simulink model "Final_project"  (R2020a)
settings: Solver=ode15s  StartTime=0.0  StopTime=1.6*3600  RelTol=1e-9
values from neighbouring files (symbols this model uses):
  a = (rp + ra)/2    (= 6781)    [final_project_data.m]
  alfa_earth = alfa_earth/alfa_tot    (= 0.0757575757576)    [final_project_data.m]
  alfa_mag = alfa_mag/alfa_tot    (= 0.0151515151515)    [final_project_data.m]
  alfa_sun = alfa_sun/alfa_tot    (= 0.454545454545)    [final_project_data.m]
  e = (ra - rp)/(rp + ra)    (= 0.00147470874502)    [final_project_data.m]
  F_e = 1358    [final_project_data.m]
  G = 6.67408e-11    [final_project_data.m]
  GK = lqr(A,B,Q,R)    [final_project_data.m]
  i = 51.6    [final_project_data.m]
  I_x = I(1)    [final_project_data.m]
  I_y = I(2)    [final_project_data.m]
  I_z = I(3)    [final_project_data.m]
  m_earth = 5.972e+24    [final_project_data.m]
  mu_e = 398600    [final_project_data.m]
  n = sqrt(mu_e/a^3)    [final_project_data.m]
  omega = 0    [final_project_data.m]
  omega_e = 2*pi/T_earth    (= 7.29212351699e-05)    [final_project_data.m]
  R_e = 6371    [final_project_data.m]
  RAAN = 0    [final_project_data.m]
undefined symbols (not defined in the file or in its folder): gm, gn, gvali, hm, hn, hvali
libraries: vrlib x4, simulink_extras x3
(part 1 of 2)
settings Model: SimulationMode=accelerator  Creator=dvdia  LastModifiedBy=dvdia
settings SolverCC: ZeroCrossAlgorithm=Adaptive
settings DebuggingCC: ReadBeforeWriteMsg=DisableAll  WriteAfterWriteMsg=DisableAll  WriteAfterReadMsg=DisableAll  IgnoredZcDiagnostic=none  MultiTaskDSMMsg=none
settings ModelReferenceCC: UpdateModelReferenceTargets=IfOutOfDate
settings SFSimCC: SFSimEcho=off  CustomCodeUndefinedFunction=UseInterfaceOnly

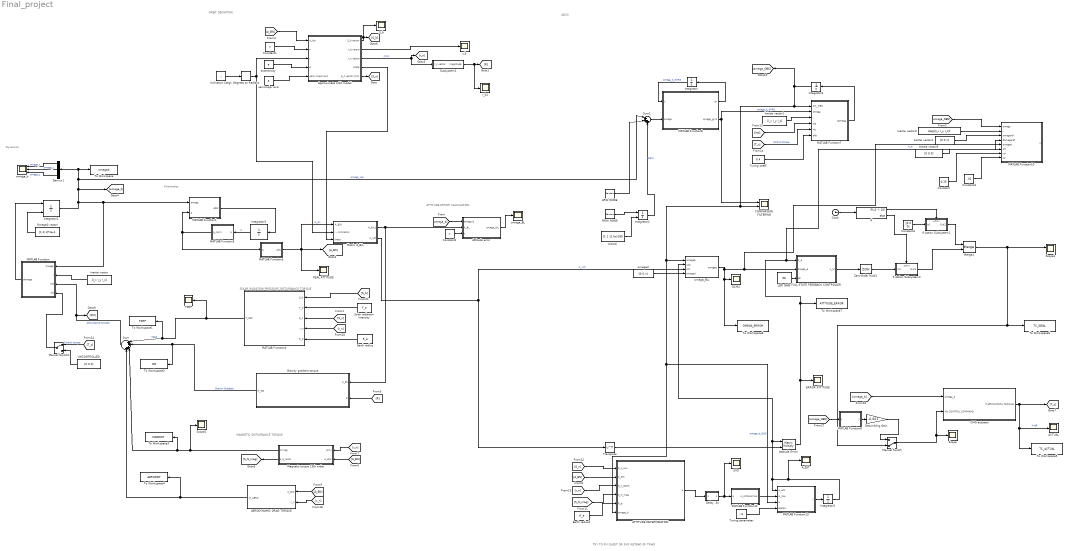
== system Final_project ==
  note: TRY TO FIX QUEST OR SVD INSTEAD OF TRIAD
  note: ADCS
  note: MAGNETIC DISTURBANCE TORQUE
  note: SOLAR RADIATION PRESSURE DISTURBANCE TORQUE
  note: ORBIT DEFINITION
  note: ATTITUDE ERROR CALCULATION
  note: Kinematics
  note: Dynamics
  ACTUAL : Scope
  AERODYNAMIC DRAG TORQUE : Subsystem
  ARW NOISE : RandomNumber  Variance=(0.0025*pi/180).^2.*[1 1 1]  SampleTime=1/10
  ATTITUDE DETERMINATION : Subsystem
  A_EST : Scope
  Approximate orbit model : Subsystem
  Attitude Errror : Product  Multiplication=Matrix(*)
  Attitude error : Subsystem
  CMG actuator : Subsystem
  COMPARISON FILTERING : Scope  NumInputPorts=2
  Clock : Clock
  Constant : Constant  Value=0.25
  Constant1 : Constant  Value=n
  Constant2 : Constant  Value=n
  Constant3 : Constant  Value=.01
  Constant4 : Constant  Value=[0 0 0]
  DCM2 : Scope
  Degrees to Radians : simulink_extras/Transformations/Degrees to Radians
  Delay .5s : Subsystem
  Demux1 : Demux  Outputs=3
  Detumbling Gain : Gain  Gain=-0.001
  ERROR ATTITUDE : Scope
  Earth radius : Constant  Value=R_e
  Earth radius1 : Constant  Value=R_e
  FULL STATE FEEDBACK CONTROLLER : MATLAB Function  TreatAsAtomicUnit=on
  Gravity gradient torque : Subsystem
  If : If  IfExpression=u1 < 10
  If Action Subsystem1 : Subsystem  TreatAsAtomicUnit=on
  If Action Subsystem2 : Subsystem  TreatAsAtomicUnit=on
  Inertia vector : Constant  Description=Inertia vector containing the inertias of the spacecraft in a PRINCIPAL AXIS REFERENCE SYSTEM  Value=[I_x I_y I_z]
  Inertia vector1 : Constant  Description=Inertia vector containing the inertias of the spacecraft in a PRINCIPAL AXIS REFERENCE SYSTEM  Value=[I_x I_y I_z]
  Inertia vector3 : Constant  Description=Inertia vector containing the inertias of the spacecraft in a PRINCIPAL AXIS REFERENCE SYSTEM  Value=diag([I_x I_y I_z])
  Inertia vector4 : Constant  Description=Inertia vector containing the inertias of the spacecraft in a PRINCIPAL AXIS REFERENCE SYSTEM  Value=[0 0 n]
  Inertia vector5 : Constant  Description=Inertia vector containing the inertias of the spacecraft in a PRINCIPAL AXIS REFERENCE SYSTEM  Value=[0 0 0]
  Integrator : Integrator  InitialCondition=[0 0 0 0 0 0]
  Integrator1 : Integrator  InitialConditionSource=external  InitialCondition=[1e-6 1e-6 n]
  Integrator2 : Integrator  InitialConditionSource=external  InitialCondition=[1 1 1].*
  Integrator3 : Integrator  InitialCondition=[ 0 0 0 1]
  Integrator4 : Integrator  InitialCondition=[0 0 0]
  Integrator5 : Integrator  InitialCondition=eye(3)
  LQR GAIN : Constant  Value=GK
  MATLAB Function : MATLAB Function  TreatAsAtomicUnit=on
  MATLAB Function1 : MATLAB Function  TreatAsAtomicUnit=on
  MATLAB Function10 : MATLAB Function  TreatAsAtomicUnit=on
  MATLAB Function11 : MATLAB Function  TreatAsAtomicUnit=on
  MATLAB Function13 : MATLAB Function  TreatAsAtomicUnit=on
  MATLAB Function3 : MATLAB Function  TreatAsAtomicUnit=on
  MATLAB Function4 : MATLAB Function  TreatAsAtomicUnit=on
  MATLAB Function5 : MATLAB Function  TreatAsAtomicUnit=on
  MATLAB Function6 : MATLAB Function  TreatAsAtomicUnit=on
  MATLAB Function7 : MATLAB Function  TreatAsAtomicUnit=on
  MATLAB Function8 : MATLAB Function  TreatAsAtomicUnit=on
  Magnetic torque 13th order : Subsystem
  Manual Switch : ManualSwitch  CurrentSetting=0
  Manual Switch1 : ManualSwitch
  Matrix A_B/L : Subsystem
  Merge1 : Merge
  Omega0 vector : Constant  Description=Inertia vector containing the inertias of the spacecraft in a PRINCIPAL AXIS REFERENCE SYSTEM  Value=[1;1;1]*1e-1
  REAL ATTITUDE : Scope
  "RRW NOISE " : RandomNumber  Variance=(1.5e-8*pi/180).^2.*[1 1 1]  SampleTime=1/10
  SVD : Scope
  S_b : Scope
  Scope : Scope
  Scope1 : Scope  NumInputPorts=2
  Scope2 : Scope
  Solar radiation intensity : Constant  Value=F_e
  Subsystem1 : Subsystem
  Sum : Sum  Inputs=|++++
  Sum1 : Sum  Inputs=|+++
  TSRP : Scope
  To Workspace : ToWorkspace  VariableName=omegab  SaveFormat=Timeseries  SampleTime=-1
  To Workspace1 : ToWorkspace  VariableName=TSRP  SaveFormat=Timeseries  SampleTime=-1
  To Workspace2 : ToWorkspace  VariableName=GG  SaveFormat=Timeseries  SampleTime=-1
  To Workspace3 : ToWorkspace  VariableName=MAGDIST  SaveFormat=Timeseries  SampleTime=-1
  To Workspace4 : ToWorkspace  VariableName=AERODIST  SaveFormat=Timeseries  SampleTime=-1
  To Workspace5 : ToWorkspace  VariableName=TC_ACTUAL  SaveFormat=Timeseries  SampleTime=-1
  To Workspace6 : ToWorkspace  VariableName=TC_IDEAL  SaveFormat=Timeseries  SampleTime=-1
  To Workspace7 : ToWorkspace  VariableName=ATTITUDE_ERROR  SaveFormat=Timeseries  SampleTime=-1
  To Workspace8 : ToWorkspace  VariableName=OMEGA_ERROR  SaveFormat=Timeseries  SampleTime=-1
  Transpose : Math  Operator=transpose  SaturateOnIntegerOverflow=on
  Tuning coeff. : Constant  Description=Inertia vector containing the inertias of the spacecraft in a PRINCIPAL AXIS REFERENCE SYSTEM  Value=0.4
  Tuning parameter : Constant  Value=-.6
  UNCONTROLLED : Constant  Description=Inertia vector containing the inertias of the spacecraft in a PRINCIPAL AXIS REFERENCE SYSTEM  Value=[0 0 0]
  Zero-Order Hold1 : ZeroOrderHold  SampleTime=-1
  b(t=0) : Constant  Value=[1 1 1].*pi/180
  eccentricity : Constant  Value=e
  inclination [deg] : Constant  Value=i
  omega_BL : Scope
  omega_B\L : MATLAB Function  TreatAsAtomicUnit=on
  omega_b : Scope  NumInputPorts=3
  omegad : Constant  Description=Inertia vector containing the inertias of the spacecraft in a PRINCIPAL AXIS REFERENCE SYSTEM  Value=[0 0 n]
  r_b : Scope
  r_b1 : Scope
  semimajor axis : Constant  Value=a
  wires:
  Demux1/1 -> omega_b/1  "omega_x"
  Demux1/2 -> omega_b/2  "omega_y"
  MATLAB Function/1(domega) -> Integrator1/1
  Demux1/3 -> omega_b/3  "omega_z"
  Inertia vector/1 -> MATLAB Function/2(I)
  Matrix A_B/L/1(A_B/L1) -> Gravity gradient torque/1(A_BL), Attitude error/2(A_BL)
  inclination [deg]/1 -> Degrees to Radians/1
  Degrees to Radians/1 -> Approximate orbit model/3(" i"), Matrix A_B/L/2(i - inclination)
  Approximate orbit model/4(theta) -> Matrix A_B/L/3(theta)
  eccentricity/1 -> Approximate orbit model/4(" e")
  Constant1/1 -> Approximate orbit model/2("n ")
  [A_BN] -> Approximate orbit model/1(A_b/n)
  semimajor axis/1 -> Approximate orbit model/5(" semi-major axis")
  Approximate orbit model/2(r_b versor) -> r_b/1
  Solar radiation intensity/1 -> MATLAB Function4/2(F_e)
  MATLAB Function4/1(T_SRP) -> To Workspace1/1, Sum/1, TSRP/1  "TSRP"
  Earth radius/1 -> MATLAB Function4/5(R_e)
  Subsystem1/1(magnitude) -> r_b1/1, [R]
  [R] -> Gravity gradient torque/2(R)
  Constant2/1 -> Attitude error/3(n)
  Attitude error/1(omega_B/L) -> omega_BL/1
  Sum/1 -> MATLAB Function/3(Md), [Md]  "Disturbance torques"
  [A_BN] -> Magnetic torque 13th order/2(A_B/N)
  [r_n] -> Magnetic torque 13th order/1("[km]")
  MATLAB Function5/1(q_norm) -> MATLAB Function1/2(q), MATLAB Function3/1(q)
  Integrator1/1 -> Demux1/1, To Workspace/1, Sum1/1, [omega_b], MATLAB Function/1(omega), MATLAB Function1/1(omega)  "omega_vec"
  Integrator3/1 -> MATLAB Function5/1(q)  "q"
  MATLAB Function1/1(qdot) -> Integrator3/1
  MATLAB Function3/1(Abn) -> REAL ATTITUDE/1, [A_BN], Matrix A_B/L/1(A_B/N)  "A_bn"
  [omega_b] -> CMG actuator/1(omega_b)
  CMG actuator/1(M eff CONTROL TORQUE) -> [T_c], To Workspace5/1, ACTUAL/1  "M eff"
  Magnetic torque 13th order/2(b_N_MAG) -> [S_N_mag]
  Omega0 vector/1 -> Integrator1/2
  Approximate orbit model/3(r_n vector) -> [r_n], Subsystem1/1(r_n vector)  "[km]"
  [r_n] -> MATLAB Function4/4(r_n)
  Approximate orbit model/1(S_b versor) -> S_b/1, [S_b]
  [S_b] -> MATLAB Function4/1(S_b)
  [S_n] -> MATLAB Function4/3(S_n)
  Approximate orbit model/5(S_n vector [km]) -> [S_n]
  [A_BN] -> AERODYNAMIC DRAG TORQUE/1(A_B/N)
  [r_n] -> AERODYNAMIC DRAG TORQUE/2(r_n)
  AERODYNAMIC DRAG TORQUE/1(M_AERO) -> To Workspace4/1, Sum/4
  Magnetic torque 13th order/1(M mag) -> Scope2/1, To Workspace3/1, Sum/3
  Gravity gradient torque/1(M_GG) -> To Workspace2/1, Sum/2  "Gravity Gradient"
  [omega_OBS] -> MATLAB Function6/1(u)
  MATLAB Function6/1(y) -> Detumbling Gain/1
  Merge1/1 -> Scope1/1, Manual Switch/2, To Workspace6/1
  [S_n] -> ATTITUDE DETERMINATION/1(S_n_sun)
  [A_BN] -> ATTITUDE DETERMINATION/2(A_BN)
  [r_n] -> ATTITUDE DETERMINATION/3(S_n_earth)
  [S_N_mag] -> ATTITUDE DETERMINATION/4(S_N_mag)
  Matrix A_B/L/2(A_L/N) -> omega_B\L/3(Aln), Transpose/1  "A_L/N"
  Transpose/1 -> Attitude Errror/2
  Attitude Errror/1 -> MATLAB Function10/6(Ae), FULL STATE FEEDBACK CONTROLLER/1(A_e), To Workspace7/1, ERROR ATTITUDE/1  "A_e"
  Integrator/1 -> MATLAB Function8/1(x)  "omega_b_GYRO"
  MATLAB Function8/1(dx) -> Integrator/1
  MATLAB Function8/2(omega_gyro) -> MATLAB Function7/2(omega), COMPARISON FILTERING/1  "omega_b_GYRO"
  Sum1/1 -> MATLAB Function8/2(omega)
  "RRW NOISE "/1 -> Integrator2/1
  Integrator2/1 -> Sum1/3  "RRW"
  b(t=0)/1 -> Integrator2/2
  ARW NOISE/1 -> Sum1/2
  Inertia vector1/1 -> MATLAB Function7/3(I)
  Integrator4/1 -> [omega_OBS], COMPARISON FILTERING/2, omega_B\L/1(omegab), ATTITUDE DETERMINATION/6(omega_b), MATLAB Function13/3(w), MATLAB Function7/1(om_OBS)  "omega_b_OBS"
  MATLAB Function7/1(domega) -> Integrator4/1
  [T_c] -> MATLAB Function7/5(Mc)  "Control torque"
  [Md] -> MATLAB Function7/4(Md)
  Tuning coeff./1 -> MATLAB Function7/6(alfa)
  Manual Switch/1 -> Scope/1, CMG actuator/2(Mc CONTROL COMMAND)
  Clock/1 -> If/1
  Constant4/1 -> If Action Subsystem1/1(In1)
  If/1 -> If Action Subsystem1/Action
  If/2 -> If Action Subsystem2/Action
  If Action Subsystem1/1(Out1) -> Merge1/1
  If Action Subsystem2/1(Out1) -> Merge1/2
  Tuning parameter/1 -> MATLAB Function13/4(alpha1)
  MATLAB Function13/1(y) -> Integrator5/1
  Detumbling Gain/1 -> Manual Switch/1
  omegad/1 -> omega_B\L/4(omegad)
  MATLAB Function11/1(A_orthonormal) -> MATLAB Function13/2(A_raw)
  FULL STATE FEEDBACK CONTROLLER/1(u_id) -> Zero-Order Hold1/1
  LQR GAIN/1 -> FULL STATE FEEDBACK CONTROLLER/3(GK)
  Delay .5s/1(Out1) -> SVD/1, MATLAB Function11/1(A)
  ATTITUDE DETERMINATION/1(A) -> Delay .5s/1(In1)
  Earth radius1/1 -> ATTITUDE DETERMINATION/5(R_e)
  Integrator5/1 -> A_EST/1, omega_B\L/2(Abn), Attitude Errror/1, MATLAB Function13/1(A_est)
  Manual Switch1/1 -> MATLAB Function/4(Mc)
  [T_c] -> Manual Switch1/1  "Control torque"
  UNCONTROLLED/1 -> Manual Switch1/2
  [omega_b] -> Attitude error/1(omega_b)
  Inertia vector3/1 -> MATLAB Function10/2(J)
  Constant/1 -> MATLAB Function10/7(kd)
  Inertia vector5/1 -> MATLAB Function10/4(domegaref)
  Constant3/1 -> MATLAB Function10/8(kp)
  Inertia vector4/1 -> MATLAB Function10/3(omegaref)
  omega_B\L/1(omegae) -> To Workspace8/1, DCM2/1, MATLAB Function10/5(omegae), FULL STATE FEEDBACK CONTROLLER/2(omega_e)
  [omega_OBS] -> MATLAB Function10/1(omega)
  Zero-Order Hold1/1 -> If Action Subsystem2/1(In1)

== system Final_project/AERODYNAMIC DRAG TORQUE ==
  A_B/N : Inport
  r_n : Inport  Port=2
  "Atmosphere rotation (with Earth) " : Constant  Value=omega_e*[0;0;1]
  Cross Product : vrlib/Utilities/Cross Product
  Derivative : Derivative
  MATLAB Function6 : MATLAB Function  TreatAsAtomicUnit=on
  Product : Product  Multiplication=Matrix(*)
  Sum1 : Sum  Inputs=|++
  rho : Constant  Value=2.82*10^-14
  M_AERO : Outport
  wires:
  Derivative/1 -> Sum1/1  "v_n"
  Sum1/1 -> Product/2  "v_rel_N"
  A_B/N/1 -> Product/1
  MATLAB Function6/1(M_AERO) -> M_AERO/1
  Product/1 -> MATLAB Function6/1(v_rel_b)  "v_rel _b"
  rho/1 -> MATLAB Function6/2(rho)
  r_n/1 -> Cross Product/2, Derivative/1
  Cross Product/1 -> Sum1/2
  "Atmosphere rotation (with Earth) "/1 -> Cross Product/1

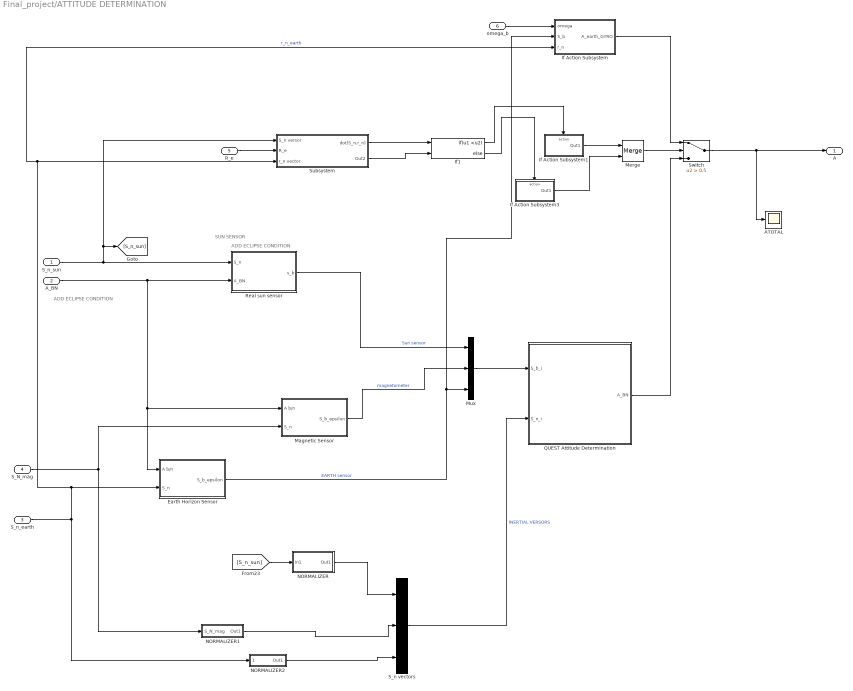
== system Final_project/ATTITUDE DETERMINATION ==
  note: ADD ECLIPSE CONDITION
  note: SUN SENSOR
  note: ADD ECLIPSE CONDITION
  S_n_sun : Inport
  A_BN : Inport  Port=2
  S_n_earth : Inport  Port=3
  S_N_mag : Inport  Port=4
  R_e : Inport  Port=5
  omega_b : Inport  Port=6
  ATOTAL : Scope
  Earth Horizon Sensor : Subsystem
  If Action Subsystem : Subsystem  TreatAsAtomicUnit=on
  If Action Subsystem1 : Subsystem  TreatAsAtomicUnit=on
  If Action Subsystem3 : Subsystem  TreatAsAtomicUnit=on
  If1 : If  NumInputs=2  IfExpression=u1 <u2
  Magnetic Sensor : Subsystem
  Merge : Merge
  Mux : Mux  Inputs=3
  NORMALIZER : Subsystem
  NORMALIZER1 : Subsystem
  NORMALIZER2 : Subsystem
  QUEST Attitude Determination : Subsystem  mask{QUEST=QUEST}
  Real sun sensor : Subsystem
  S_n vectors : Mux  Inputs=3
  Subsystem : Subsystem
  Switch : Switch  Criteria=u2 > Threshold  Threshold=0.5
  A : Outport
  wires:
  Real sun sensor/1(s_b) -> Mux/1  "Sun sensor"
  Mux/1 -> QUEST Attitude Determination/1(S_b_i)
  Magnetic Sensor/1(S_b_epsilon) -> Mux/2  "magnetometer"
  NORMALIZER/1(Out1) -> S_n vectors/1
  S_n vectors/1 -> QUEST Attitude Determination/2(S_n_i)  "INERTIAL VERSORS"
  S_N_mag/1 -> NORMALIZER1/1(S_N_mag), Magnetic Sensor/2(S_n)
  S_n_earth/1 -> NORMALIZER2/1(S_n_earth), If Action Subsystem/3(r_n), Subsystem/3(r_n vector), Earth Horizon Sensor/2(S_n)  "r_n_earth"
  [S_n_sun] -> NORMALIZER/1(In1)
  A_BN/1 -> Real sun sensor/2(A_BN), Magnetic Sensor/1(A b/n), Earth Horizon Sensor/1(A b/n)
  S_n_sun/1 -> [S_n_sun], Subsystem/1(S_n versor), Real sun sensor/1(S_n)
  Earth Horizon Sensor/1(S_b_epsilon) -> Mux/3, If Action Subsystem/2(S_b)  "EARTH sensor"
  NORMALIZER1/1(Out1) -> S_n vectors/2
  NORMALIZER2/1(Out1) -> S_n vectors/3
  QUEST Attitude Determination/1(A_BN) -> Switch/3
  Switch/1 -> A/1, ATOTAL/1
  If Action Subsystem/1(A_earth_GYRO) -> Switch/1
  If1/2 -> If Action Subsystem3/Action
  R_e/1 -> Subsystem/2(R_e)
  Subsystem/1(dot(S_n,r_n)) -> If1/1
  Subsystem/2(Out2) -> If1/2
  omega_b/1 -> If Action Subsystem/1(omega)
  If1/1 -> If Action Subsystem1/Action
  Merge/1 -> Switch/2
  If Action Subsystem1/1(Out1) -> Merge/1
  If Action Subsystem3/1(Out1) -> Merge/2

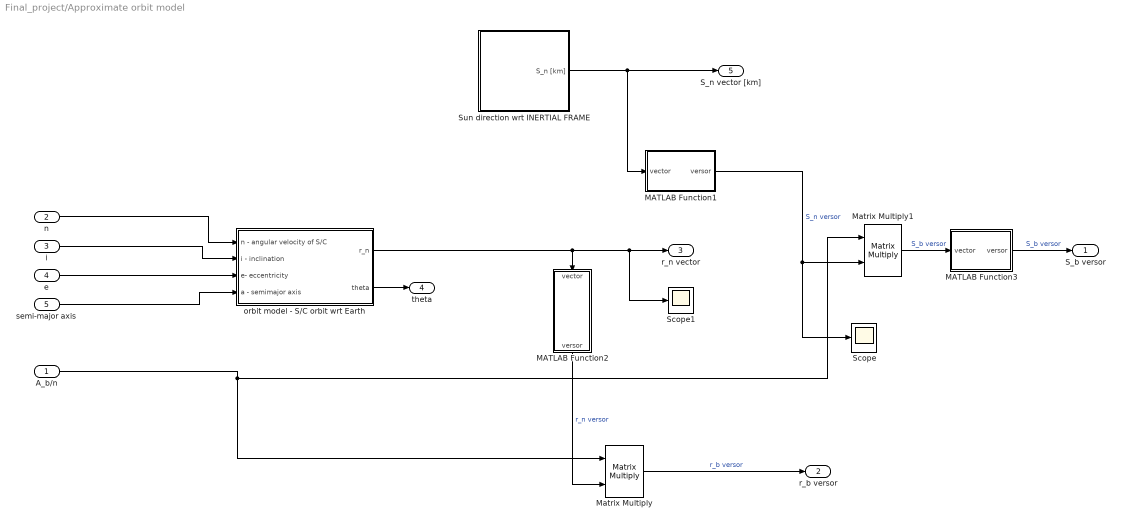
== system Final_project/Approximate orbit model ==
  A_b/n : Inport
  "n " : Inport  Port=2
  " i" : Inport  Port=3
  " e" : Inport  Port=4
  " semi-major axis" : Inport  Port=5
  MATLAB Function1 : MATLAB Function  TreatAsAtomicUnit=on
  MATLAB Function2 : MATLAB Function  TreatAsAtomicUnit=on
  MATLAB Function3 : MATLAB Function  TreatAsAtomicUnit=on
  Matrix Multiply : Product  Multiplication=Matrix(*)
  Matrix Multiply1 : Product  Multiplication=Matrix(*)
  Scope : Scope
  Scope1 : Scope
  Sun direction wrt INERTIAL FRAME : Subsystem
  orbit model - S/C orbit wrt Earth : Subsystem
  S_b versor : Outport
  r_b versor : Outport  Port=2
  r_n vector : Outport  Port=3
  theta : Outport  Port=4
  S_n vector [km] : Outport  Port=5
  wires:
  orbit model - S/C orbit wrt Earth/1(r_n) -> MATLAB Function2/1(vector), Scope1/1, r_n vector/1
  MATLAB Function1/1(versor) -> Scope/1, Matrix Multiply1/2  "S_n versor"
  A_b/n/1 -> Matrix Multiply/1, Matrix Multiply1/1
  MATLAB Function2/1(versor) -> Matrix Multiply/2  "r_n versor"
  Sun direction wrt INERTIAL FRAME/1(S_n [km]) -> S_n vector [km]/1, MATLAB Function1/1(vector)
  "n "/1 -> orbit model - S/C orbit wrt Earth/1(n - angular velocity of S/C)
  " i"/1 -> orbit model - S/C orbit wrt Earth/2(i - inclination)
  " e"/1 -> orbit model - S/C orbit wrt Earth/3(e- eccentricity)
  Matrix Multiply/1 -> r_b versor/1  "r_b versor"
  orbit model - S/C orbit wrt Earth/2(theta) -> theta/1
  " semi-major axis"/1 -> orbit model - S/C orbit wrt Earth/4(a - semimajor axis)
  MATLAB Function3/1(versor) -> S_b versor/1  "S_b versor"
  Matrix Multiply1/1 -> MATLAB Function3/1(vector)  "S_b versor"

== system Final_project/Attitude error ==
  omega_b : Inport
  A_BL : Inport  Port=2
  n : Inport  Port=3
  " " : Product  Multiplication=Matrix(*)
  Sum : Sum  Inputs=|-+
  omega_L/N : Subsystem
  omega_B/L : Outport
  wires:
  Sum/1 -> omega_B/L/1  "omega_B/L"
  omega_L/N/1(omega_L/N) -> " "/2
  " "/1 -> Sum/1
  omega_b/1 -> Sum/2
  A_BL/1 -> " "/1
  n/1 -> omega_L/N/1(omega z)

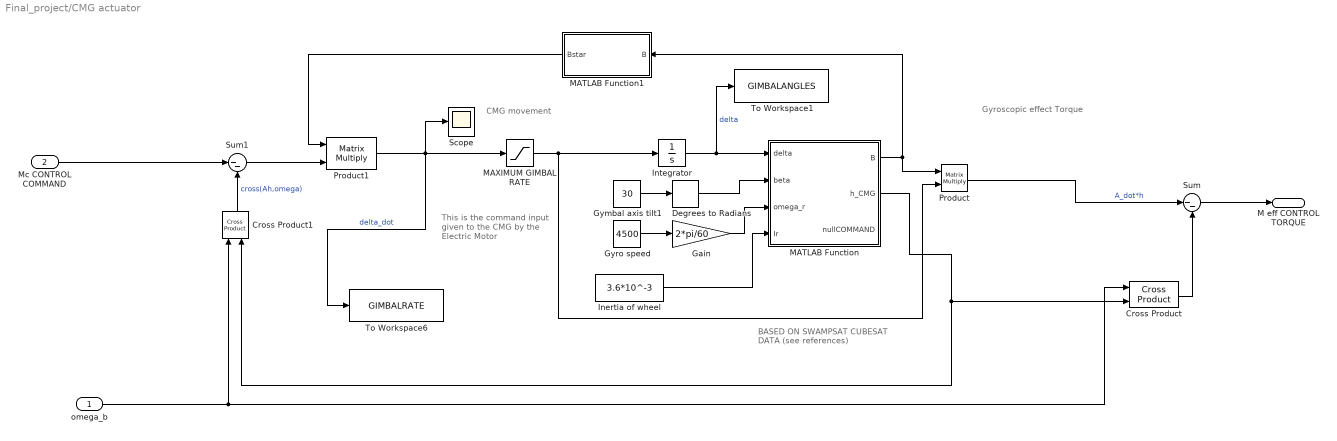
== system Final_project/CMG actuator ==
  note: BASED ON SWAMPSAT
      | CUBESAT DATA (see references)
  note: Gyroscopic effect Torque
  note: CMG movement
  note: This is the command input given to the
      | CMG by the Electric Motor
  omega_b : Inport
  Mc CONTROL COMMAND : Inport  Port=2
  Cross Product : vrlib/Utilities/Cross Product
  Cross Product1 : vrlib/Utilities/Cross Product
  Degrees to Radians : simulink_extras/Transformations/Degrees to Radians
  Gain : Gain  Gain=2*pi/60
  Gymbal axis tilt1 : Constant  Value=30
  Gyro speed : Constant  Value=4500
  Inertia of wheel : Constant  Value=3.6*10^-3
  Integrator : Integrator  InitialCondition=[0 0 0 0]
  MATLAB Function : MATLAB Function  TreatAsAtomicUnit=on
  MATLAB Function1 : MATLAB Function  TreatAsAtomicUnit=on
  MAXIMUM GIMBAL RATE : Saturate  UpperLimit=1  LowerLimit=-1
  Product : Product  Multiplication=Matrix(*)
  Product1 : Product  Multiplication=Matrix(*)
  Scope : Scope
  Sum : Sum  Inputs=|--
  Sum1 : Sum  Inputs=|--
  To Workspace1 : ToWorkspace  VariableName=GIMBALANGLES  SaveFormat=Timeseries  SampleTime=-1
  To Workspace6 : ToWorkspace  VariableName=GIMBALRATE  SaveFormat=Timeseries  SampleTime=-1
  M eff CONTROL TORQUE : Outport
  wires:
  Integrator/1 -> To Workspace1/1, MATLAB Function/1(delta)  "delta"
  Gymbal axis tilt1/1 -> Degrees to Radians/1
  Degrees to Radians/1 -> MATLAB Function/2(beta)
  Gyro speed/1 -> Gain/1
  Gain/1 -> MATLAB Function/3(omega_r)
  Inertia of wheel/1 -> MATLAB Function/4(Ir)
  Product/1 -> Sum/1  "A_dot*h"
  omega_b/1 -> Cross Product/1, Cross Product1/1
  Cross Product/1 -> Sum/2
  Sum/1 -> M eff CONTROL TORQUE/1
  MATLAB Function1/1(Bstar) -> Product1/1
  Mc CONTROL COMMAND/1 -> Sum1/1
  Sum1/1 -> Product1/2
  Cross Product1/1 -> Sum1/2  "cross(Ah,omega)"
  MAXIMUM GIMBAL RATE/1 -> Integrator/1, Product/2
  MATLAB Function/1(B) -> Product/1, MATLAB Function1/1(B)
  MATLAB Function/2(h_CMG) -> Cross Product/2, Cross Product1/2
  Product1/1 -> To Workspace6/1, MAXIMUM GIMBAL RATE/1, Scope/1  "delta_dot"

== system Final_project/Delay .5s ==
  In1 : Inport
  Clock1 : Clock
  Constant6 : Constant  Value=ones(3)
  If Action Subsystem3 : Subsystem  TreatAsAtomicUnit=on
  If Action Subsystem4 : Subsystem  TreatAsAtomicUnit=on
  If1 : If  IfExpression=u1 < 0.5
  Merge2 : Merge
  Out1 : Outport
  wires:
  If1/1 -> If Action Subsystem3/Action
  Merge2/1 -> Out1/1
  If1/2 -> If Action Subsystem4/Action
  If Action Subsystem4/1(Out1) -> Merge2/2
  If Action Subsystem3/1(Out1) -> Merge2/1
  Constant6/1 -> If Action Subsystem3/1(In1)
  In1/1 -> If Action Subsystem4/1(In1)
  Clock1/1 -> If1/1

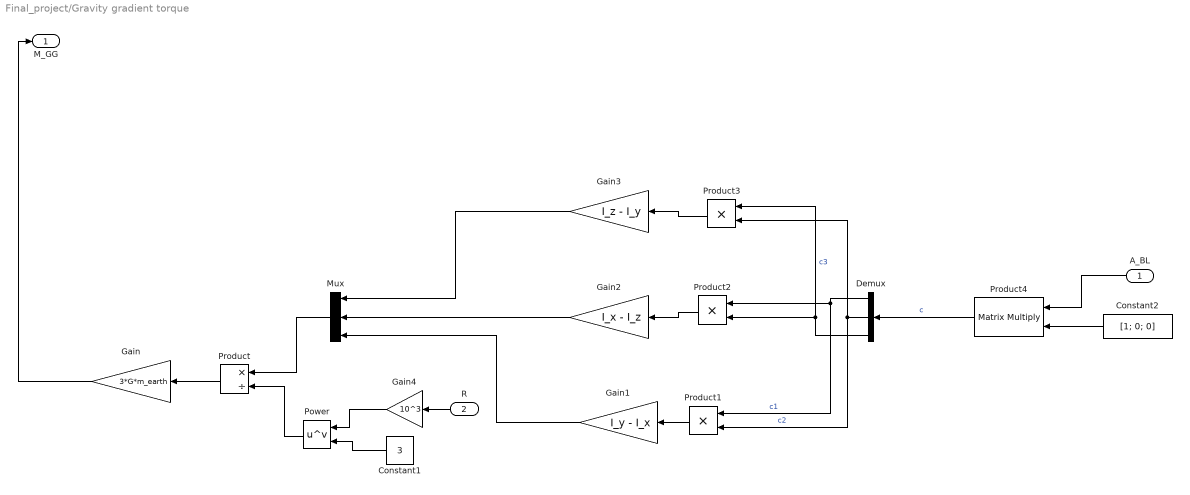
== system Final_project/Gravity gradient torque ==
  A_BL : Inport
  R : Inport  Port=2
  Constant1 : Constant  Value=3
  Constant2 : Constant  Value=[1; 0; 0]
  Demux : Demux  Outputs=3
  Gain : Gain  Gain=3*G*m_earth
  Gain1 : Gain  Gain=I_y - I_x
  Gain2 : Gain  Gain=I_x - I_z
  Gain3 : Gain  Gain=I_z - I_y
  Gain4 : Gain  Gain=10^3
  Mux : Mux  Inputs=3
  Power : Math  Operator=pow  SaturateOnIntegerOverflow=on
  Product : Product  Inputs=*/
  Product1 : Product
  Product2 : Product
  Product3 : Product
  Product4 : Product  Multiplication=Matrix(*)
  M_GG : Outport
  wires:
  Constant1/1 -> Power/2
  Gain4/1 -> Power/1
  Demux/1 -> Product1/1, Product2/1  "c1"
  Power/1 -> Product/2
  Product/1 -> Gain/1
  Gain3/1 -> Mux/1
  Constant2/1 -> Product4/2
  Product1/1 -> Gain1/1
  Demux/2 -> Product1/2, Product3/2  "c2"
  Product3/1 -> Gain3/1
  Gain1/1 -> Mux/3
  Gain/1 -> M_GG/1
  Product4/1 -> Demux/1  "c"
  R/1 -> Gain4/1
  Mux/1 -> Product/1
  Product2/1 -> Gain2/1
  Gain2/1 -> Mux/2
  Demux/3 -> Product2/2, Product3/1  "c3"
  A_BL/1 -> Product4/1

== system Final_project/If Action Subsystem1 ==
  In1 : Inport
  Action Port : ActionPort  ActionPortLabel=if(u1 < 10)
  Out1 : Outport
  wires:
  In1/1 -> Out1/1

== system Final_project/If Action Subsystem2 ==
  In1 : Inport
  Action Port : ActionPort  ActionPortLabel=else
  Out1 : Outport
  wires:
  In1/1 -> Out1/1

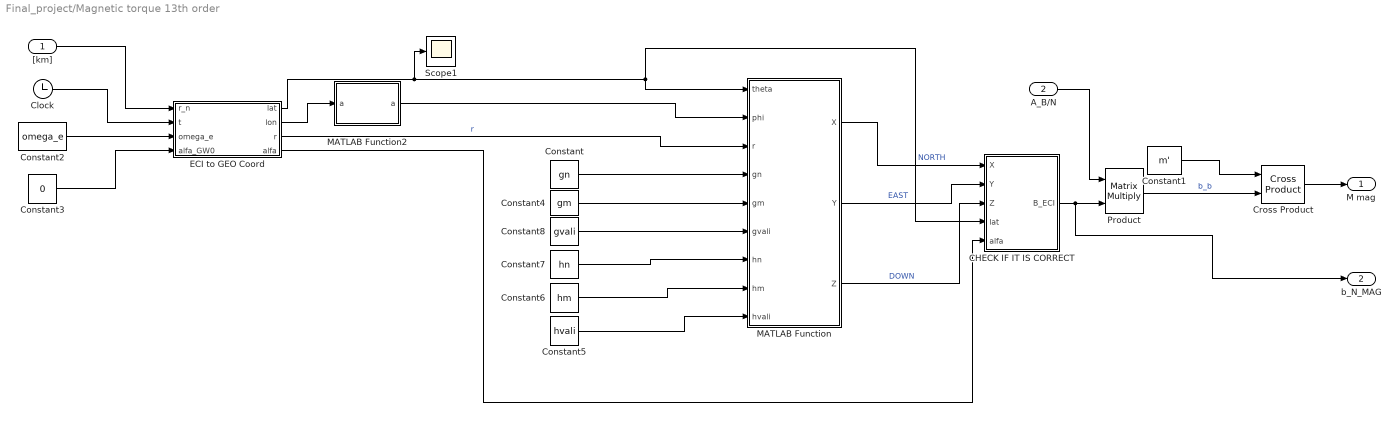
== system Final_project/Magnetic torque 13th order ==
  "[km]" : Inport
  A_B/N : Inport  Port=2
  CHECK IF IT IS CORRECT : MATLAB Function  TreatAsAtomicUnit=on
  Clock : Clock
  Constant : Constant  Value=gn
  Constant1 : Constant  Value=m'
  Constant2 : Constant  Value=omega_e
  Constant3 : Constant  Value=0
  Constant4 : Constant  Value=gm
  Constant5 : Constant  Value=hvali
  Constant6 : Constant  Value=hm
  Constant7 : Constant  Value=hn
  Constant8 : Constant  Value=gvali
  Cross Product : vrlib/Utilities/Cross Product
  ECI to GEO Coord : MATLAB Function  TreatAsAtomicUnit=on
  MATLAB Function : MATLAB Function  TreatAsAtomicUnit=on
  MATLAB Function2 : MATLAB Function  TreatAsAtomicUnit=on
  Product : Product  Multiplication=Matrix(*)
  Scope1 : Scope
  M mag : Outport
  b_N_MAG : Outport  Port=2
  wires:
  Constant3/1 -> ECI to GEO Coord/4(alfa_GW0)
  ECI to GEO Coord/1(lat) -> Scope1/1, CHECK IF IT IS CORRECT/4(lat), MATLAB Function/1(theta)
  Clock/1 -> ECI to GEO Coord/2(t)
  Constant2/1 -> ECI to GEO Coord/3(omega_e)
  "[km]"/1 -> ECI to GEO Coord/1(r_n)
  Cross Product/1 -> M mag/1
  Product/1 -> Cross Product/2  "b_b"
  Constant1/1 -> Cross Product/1
  A_B/N/1 -> Product/1
  Constant/1 -> MATLAB Function/4(gn)
  Constant4/1 -> MATLAB Function/5(gm)
  Constant8/1 -> MATLAB Function/6(gvali)
  Constant7/1 -> MATLAB Function/7(hn)
  Constant6/1 -> MATLAB Function/8(hm)
  Constant5/1 -> MATLAB Function/9(hvali)
  ECI to GEO Coord/3(r) -> MATLAB Function/3(r)  "r"
  MATLAB Function2/1(a) -> MATLAB Function/2(phi)
  ECI to GEO Coord/2(lon) -> MATLAB Function2/1("a ")
  ECI to GEO Coord/4(alfa) -> CHECK IF IT IS CORRECT/5(alfa)
  MATLAB Function/1(X) -> CHECK IF IT IS CORRECT/1(X)  "NORTH"
  MATLAB Function/2(Y) -> CHECK IF IT IS CORRECT/2(Y)  "EAST"
  MATLAB Function/3(Z) -> CHECK IF IT IS CORRECT/3(Z)  "DOWN"
  CHECK IF IT IS CORRECT/1(B_ECI) -> b_N_MAG/1, Product/2

== system Final_project/Matrix A_B//L ==
  note: LVLH DEFINED AS FOLLOWING:
      | - X axis toward ZENITH
      | - Y axis toward LOCAL HORIZ
      | - Z axis perpendicular to X and Y
      |   (Aligned with negative(POSITIVE??) of orbital ANG. MOM
  A_B/N : Inport
  i - inclination : Inport  Port=2
  theta : Inport  Port=3
  " " : Product  Multiplication=Matrix(*)
  Constant : Constant  Value=omega
  Constant1 : Constant  Value=RAAN
  MATLAB Function3 : MATLAB Function  TreatAsAtomicUnit=on
  Transpose : Math  Operator=transpose  SignedPower=on  SaturateOnIntegerOverflow=on
  A_B/L1 : Outport
  A_L/N : Outport  Port=2
  wires:
  MATLAB Function3/1(A_LN) -> A_L/N/1, Transpose/1
  " "/1 -> A_B/L1/1  "A_B/L"
  Transpose/1 -> " "/2
  theta/1 -> MATLAB Function3/1(theta)
  i - inclination/1 -> MATLAB Function3/2(i)
  A_B/N/1 -> " "/1
  Constant/1 -> MATLAB Function3/3(w)
  Constant1/1 -> MATLAB Function3/4(RAAN)

== system Final_project/Subsystem1 ==
  r_n vector : Inport
  Dot Product1 : DotProduct  InputSameDT=on  OutDataTypeStr=Inherit: Inherit via internal rule
  Sqrt1 : Sqrt  SaturateOnIntegerOverflow=on
  magnitude : Outport
  wires:
  Sqrt1/1 -> magnitude/1  "magnitude"
  Dot Product1/1 -> Sqrt1/1
  r_n vector/1 -> Dot Product1/1, Dot Product1/2

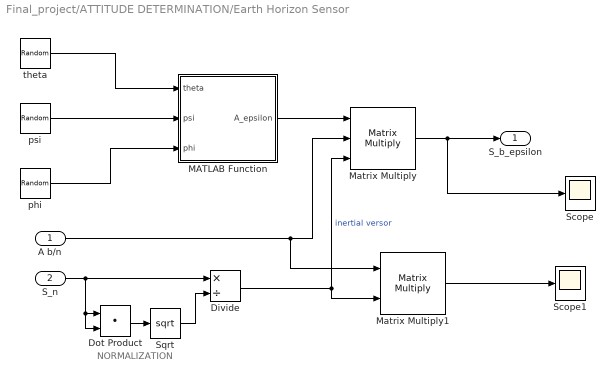
== system Final_project/ATTITUDE DETERMINATION/Earth Horizon Sensor ==
  note: NORMALIZATION
  A b/n : Inport
  S_n : Inport  Port=2
  Divide : Product  Inputs=*/
  Dot Product : DotProduct  InputSameDT=on  OutDataTypeStr=Inherit: Inherit via internal rule
  MATLAB Function : MATLAB Function  TreatAsAtomicUnit=on
  Matrix Multiply : Product  Inputs=3  Multiplication=Matrix(*)
  Matrix Multiply1 : Product  Multiplication=Matrix(*)
  Scope : Scope
  Scope1 : Scope
  Sqrt : Sqrt  SaturateOnIntegerOverflow=on
  phi : RandomNumber  Variance=deg2rad(0.1^2)  Seed=3  SampleTime=0.1
  psi : RandomNumber  Variance=deg2rad(0.1^2)  Seed=2  SampleTime=0.1
  theta : RandomNumber  Variance=deg2rad(0.1^2)  Seed=1  SampleTime=0.1
  S_b_epsilon : Outport
  wires:
  theta/1 -> MATLAB Function/1(theta)
  psi/1 -> MATLAB Function/2(psi)
  phi/1 -> MATLAB Function/3(phi)
  MATLAB Function/1(A_epsilon) -> Matrix Multiply/1
  A b/n/1 -> Matrix Multiply1/1, Matrix Multiply/2
  Divide/1 -> Matrix Multiply1/2, Matrix Multiply/3  "inertial versor"
  S_n/1 -> Divide/1, Dot Product/2, Dot Product/1
  Dot Product/1 -> Sqrt/1
  Sqrt/1 -> Divide/2
  Matrix Multiply1/1 -> Scope1/1
  Matrix Multiply/1 -> S_b_epsilon/1, Scope/1

== system Final_project/ATTITUDE DETERMINATION/If Action Subsystem ==
  omega : Inport
  S_b : Inport  Port=2
  r_n : Inport  Port=3
  Integrator6 : Integrator  InitialCondition=eye(3)
  MATLAB Function9 : MATLAB Function  TreatAsAtomicUnit=on
  A_earth_GYRO : Outport
  wires:
  MATLAB Function9/1(dA) -> Integrator6/1
  r_n/1 -> MATLAB Function9/4(r_n)
  omega/1 -> MATLAB Function9/2(w)  "omega_b_OBS"
  S_b/1 -> MATLAB Function9/3(s_b)
  Integrator6/1 -> A_earth_GYRO/1, MATLAB Function9/1(A)

== system Final_project/ATTITUDE DETERMINATION/If Action Subsystem1 ==
  Action Port : ActionPort  ActionPortLabel=if(u1 <u2)
  Constant : Constant
  Out1 : Outport
  wires:
  Constant/1 -> Out1/1

== system Final_project/ATTITUDE DETERMINATION/If Action Subsystem3 ==
  Action Port : ActionPort  ActionPortLabel=else
  Constant : Constant  Value=0
  Out1 : Outport
  wires:
  Constant/1 -> Out1/1

== system Final_project/ATTITUDE DETERMINATION/Magnetic Sensor ==
  A b/n : Inport
  S_n : Inport  Port=2
  MATLAB Function : MATLAB Function  TreatAsAtomicUnit=on
  Matrix Multiply : Product  Inputs=3  Multiplication=Matrix(*)
  NORMALIZER : Subsystem
  Scope : Scope
  phi : RandomNumber  Variance=deg2rad(0.5^2)  SampleTime=0.1
  psi : RandomNumber  Variance=deg2rad(0.5^2)  SampleTime=0.1
  theta : RandomNumber  Variance=deg2rad(0.5^2)  SampleTime=0.1
  S_b_epsilon : Outport
  wires:
  A b/n/1 -> Matrix Multiply/2
  Matrix Multiply/1 -> Scope/1, S_b_epsilon/1
  MATLAB Function/1(A_epsilon) -> Matrix Multiply/1
  phi/1 -> MATLAB Function/3(phi)
  psi/1 -> MATLAB Function/2(psi)
  theta/1 -> MATLAB Function/1(theta)
  S_n/1 -> NORMALIZER/1(In1)
  NORMALIZER/1(Out1) -> Matrix Multiply/3

== system Final_project/ATTITUDE DETERMINATION/NORMALIZER ==
  In1 : Inport
  Divide : Product  Inputs=*/
  Dot Product : DotProduct  InputSameDT=on  OutDataTypeStr=Inherit: Inherit via internal rule
  Sqrt : Sqrt  SaturateOnIntegerOverflow=on
  Out1 : Outport
  wires:
  Sqrt/1 -> Divide/2
  In1/1 -> Dot Product/1, Dot Product/2, Divide/1
  Dot Product/1 -> Sqrt/1
  Divide/1 -> Out1/1

== system Final_project/ATTITUDE DETERMINATION/NORMALIZER1 ==
  S_N_mag : Inport
  Divide : Product  Inputs=*/
  Dot Product : DotProduct  InputSameDT=on  OutDataTypeStr=Inherit: Inherit via internal rule
  Sqrt : Sqrt  SaturateOnIntegerOverflow=on
  Out1 : Outport
  wires:
  Divide/1 -> Out1/1
  Dot Product/1 -> Sqrt/1
  S_N_mag/1 -> Divide/1, Dot Product/2, Dot Product/1
  Sqrt/1 -> Divide/2

== system Final_project/ATTITUDE DETERMINATION/NORMALIZER2 ==
  S_n_earth : Inport
  Divide : Product  Inputs=*/
  Dot Product : DotProduct  InputSameDT=on  OutDataTypeStr=Inherit: Inherit via internal rule
  Sqrt : Sqrt  SaturateOnIntegerOverflow=on
  Out1 : Outport
  wires:
  Sqrt/1 -> Divide/2
  S_n_earth/1 -> Dot Product/1, Dot Product/2, Divide/1
  Dot Product/1 -> Sqrt/1
  Divide/1 -> Out1/1

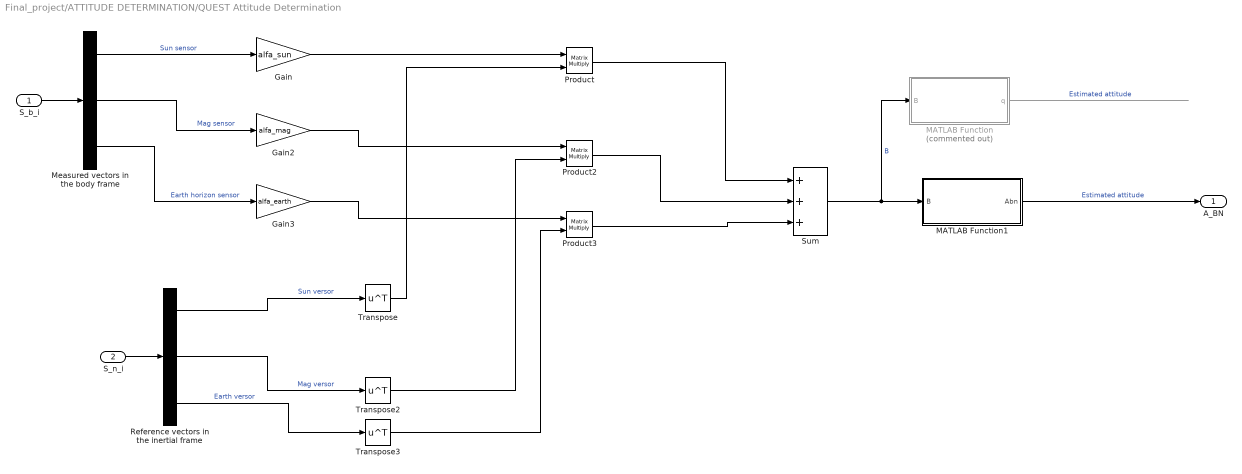
== system Final_project/ATTITUDE DETERMINATION/QUEST Attitude Determination ==
  S_b_i : Inport
  S_n_i : Inport  Port=2
  Gain : Gain  Gain=alfa_sun
  Gain2 : Gain  Gain=alfa_mag
  Gain3 : Gain  Gain=alfa_earth
  MATLAB Function : MATLAB Function  Commented=on  TreatAsAtomicUnit=on
  MATLAB Function1 : MATLAB Function  TreatAsAtomicUnit=on
  Measured vectors in the body frame : Demux  Outputs=3
  Product : Product  Multiplication=Matrix(*)
  Product2 : Product  Multiplication=Matrix(*)
  Product3 : Product  Multiplication=Matrix(*)
  Reference vectors in the inertial frame : Demux  Outputs=3
  Sum : Sum  Inputs=+++
  Transpose : Math  Operator=transpose  SaturateOnIntegerOverflow=on
  Transpose2 : Math  Operator=transpose  SaturateOnIntegerOverflow=on
  Transpose3 : Math  Operator=transpose  SaturateOnIntegerOverflow=on
  A_BN : Outport
  wires:
  S_b_i/1 -> Measured vectors in the body frame/1
  Measured vectors in the body frame/1 -> Gain/1  "Sun sensor"
  S_n_i/1 -> Reference vectors in the inertial frame/1
  Gain/1 -> Product/1
  Reference vectors in the inertial frame/1 -> Transpose/1  "Sun versor"
  Transpose/1 -> Product/2
  Product/1 -> Sum/1
  Sum/1 -> MATLAB Function1/1(B), MATLAB Function/1(B)  "B"
  MATLAB Function/1(q) -> ?  "Estimated attitude"
  Gain2/1 -> Product2/1
  Transpose2/1 -> Product2/2
  Product2/1 -> Sum/2
  Measured vectors in the body frame/3 -> Gain3/1  "Earth horizon sensor"
  Reference vectors in the inertial frame/3 -> Transpose3/1  "Earth versor"
  Gain3/1 -> Product3/1
  Transpose3/1 -> Product3/2
  Product3/1 -> Sum/3
  MATLAB Function1/1(Abn) -> A_BN/1  "Estimated attitude"
  Measured vectors in the body frame/2 -> Gain2/1  "Mag sensor"
  Reference vectors in the inertial frame/2 -> Transpose2/1  "Mag versor"

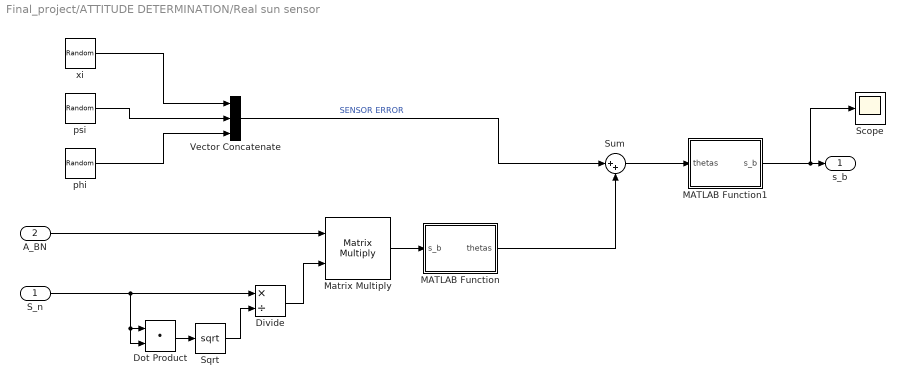
== system Final_project/ATTITUDE DETERMINATION/Real sun sensor ==
  S_n : Inport
  A_BN : Inport  Port=2
  Divide : Product  Inputs=*/
  Dot Product : DotProduct  InputSameDT=on  OutDataTypeStr=Inherit: Inherit via internal rule
  MATLAB Function : MATLAB Function  TreatAsAtomicUnit=on
  MATLAB Function1 : MATLAB Function  TreatAsAtomicUnit=on
  Matrix Multiply : Product  Multiplication=Matrix(*)
  Scope : Scope
  Sqrt : Sqrt  SaturateOnIntegerOverflow=on
  Sum : Sum  Inputs=|++
  Vector Concatenate : Concatenate  NumInputs=3
  phi : RandomNumber  Variance=deg2rad(1/6^2)  SampleTime=0.1
  psi : RandomNumber  Variance=deg2rad(1/6^2)  SampleTime=0.1
  xi : RandomNumber  Variance=deg2rad(1/6^2)  SampleTime=0.1
  s_b : Outport
  wires:
  Sqrt/1 -> Divide/2
  Divide/1 -> Matrix Multiply/2
  A_BN/1 -> Matrix Multiply/1
  S_n/1 -> Dot Product/2, Dot Product/1, Divide/1
  Dot Product/1 -> Sqrt/1
  Matrix Multiply/1 -> MATLAB Function/1(s_b)
  xi/1 -> Vector Concatenate/1
  psi/1 -> Vector Concatenate/2
  phi/1 -> Vector Concatenate/3
  Vector Concatenate/1 -> Sum/1  "SENSOR ERROR"
  MATLAB Function/1(thetas) -> Sum/2
  Sum/1 -> MATLAB Function1/1(thetas)
  MATLAB Function1/1(s_b) -> Scope/1, s_b/1

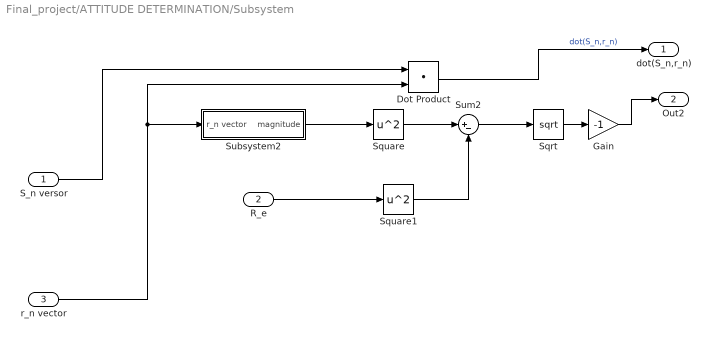
== system Final_project/ATTITUDE DETERMINATION/Subsystem ==
  S_n versor : Inport
  R_e : Inport  Port=2
  r_n vector : Inport  Port=3
  Dot Product : DotProduct  InputSameDT=on  OutDataTypeStr=Inherit: Inherit via internal rule
  Gain : Gain  Gain=-1
  Sqrt : Sqrt  SaturateOnIntegerOverflow=on
  Square : Math  Operator=square  SaturateOnIntegerOverflow=on
  Square1 : Math  Operator=square  SaturateOnIntegerOverflow=on
  Subsystem2 : Subsystem
  Sum2 : Sum  Inputs=|+-
  dot(S_n,r_n) : Outport
  Out2 : Outport  Port=2
  wires:
  r_n vector/1 -> Dot Product/2, Subsystem2/1(r_n vector)
  S_n versor/1 -> Dot Product/1
  R_e/1 -> Square1/1
  Sqrt/1 -> Gain/1
  Square/1 -> Sum2/1
  Subsystem2/1(magnitude) -> Square/1
  Square1/1 -> Sum2/2
  Sum2/1 -> Sqrt/1
  Dot Product/1 -> dot(S_n,r_n)/1  "dot(S_n,r_n)"
  Gain/1 -> Out2/1

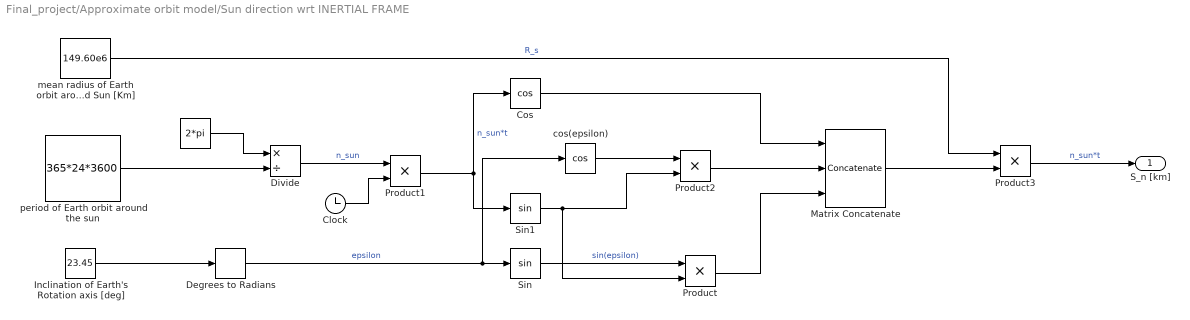
== system Final_project/Approximate orbit model/Sun direction wrt INERTIAL FRAME ==
  " " : Constant  Value=2*pi
  Clock : Clock
  Cos : Trigonometry  Operator=cos
  Degrees to Radians : simulink_extras/Transformations/Degrees to Radians
  Divide : Product  Inputs=*/
  Inclination of Earth's Rotation axis [deg] : Constant  Value=23.45
  Matrix Concatenate : Concatenate  NumInputs=3
  Product{,1..3} (4 alike) : Product  Inputs=**
  Sin : Trigonometry
  Sin1 : Trigonometry
  cos(epsilon) : Trigonometry  Operator=cos
  mean radius of Earth orbit around Sun [Km] : Constant  Value=149.60e6
  period of Earth orbit around the sun : Constant  Value=365*24*3600
  S_n [km] : Outport
  wires:
  period of Earth orbit around the sun/1 -> Divide/2
  " "/1 -> Divide/1
  Divide/1 -> Product1/1  "n_sun"
  mean radius of Earth orbit around Sun [Km]/1 -> Product3/1  "R_s"
  Inclination of Earth's Rotation axis [deg]/1 -> Degrees to Radians/1
  Degrees to Radians/1 -> Sin/1, cos(epsilon)/1  "epsilon"
  Sin/1 -> Product/1  "sin(epsilon)"
  Product1/1 -> Cos/1, Sin1/1  "n_sun*t"
  Clock/1 -> Product1/2
  Sin1/1 -> Product2/2, Product/2
  Cos/1 -> Matrix Concatenate/1
  Product/1 -> Matrix Concatenate/3
  cos(epsilon)/1 -> Product2/1
  Product2/1 -> Matrix Concatenate/2
  Matrix Concatenate/1 -> Product3/2
  Product3/1 -> S_n [km]/1  "n_sun*t"

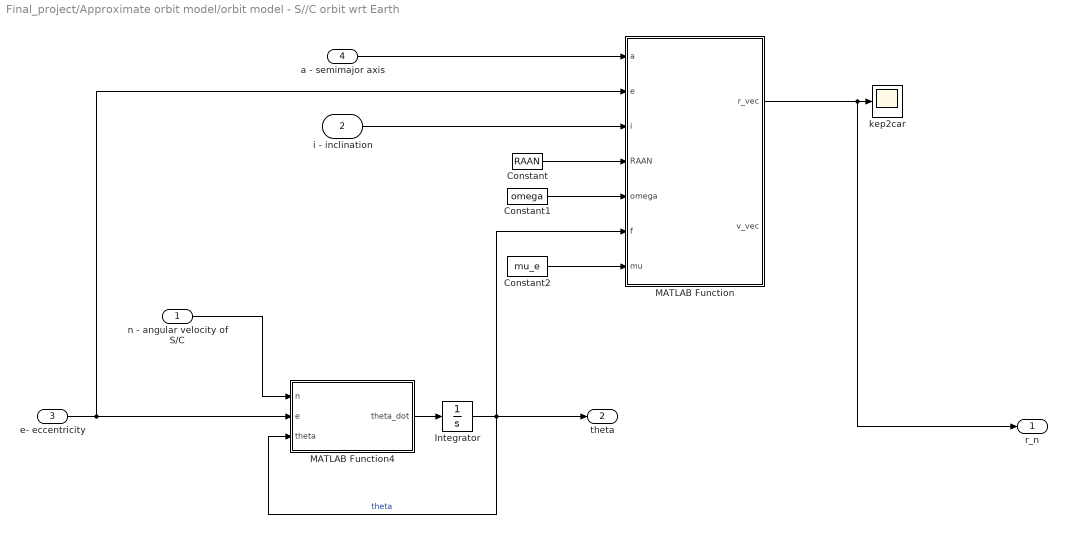
== system Final_project/Approximate orbit model/orbit model - S//C orbit wrt Earth ==
  n - angular velocity of S/C : Inport
  i - inclination : Inport  Port=2
  e- eccentricity : Inport  Port=3
  a - semimajor axis : Inport  Port=4
  Constant : Constant  Value=RAAN
  Constant1 : Constant  Value=omega
  Constant2 : Constant  Value=mu_e
  Integrator : Integrator
  MATLAB Function : MATLAB Function  TreatAsAtomicUnit=on
  MATLAB Function4 : MATLAB Function  TreatAsAtomicUnit=on
  kep2car : Scope
  r_n : Outport
  theta : Outport  Port=2
  wires:
  n - angular velocity of S/C/1 -> MATLAB Function4/1(n)
  Integrator/1 -> MATLAB Function4/3(theta), MATLAB Function/6(f), theta/1  "theta"
  MATLAB Function4/1(theta_dot) -> Integrator/1
  e- eccentricity/1 -> MATLAB Function4/2(e), MATLAB Function/2(e)
  Constant2/1 -> MATLAB Function/7(mu)
  Constant/1 -> MATLAB Function/4(RAAN)
  Constant1/1 -> MATLAB Function/5(omega)
  MATLAB Function/1(r_vec) -> r_n/1, kep2car/1
  i - inclination/1 -> MATLAB Function/3(i)
  a - semimajor axis/1 -> MATLAB Function/1(a)

== system Final_project/Attitude error/omega_L//N ==
  omega z : Inport
  Initial conditions : Concatenate  NumInputs=3  ConcatenateDimension=3
  w_x,w_y : Constant  Value=0
  omega_L/N : Outport
  wires:
  Initial conditions/1 -> omega_L/N/1  "omega"
  w_x,w_y/1 -> Initial conditions/2, Initial conditions/1  "omega_y"
  omega z/1 -> Initial conditions/3

== system Final_project/Delay .5s/If Action Subsystem3 ==
  In1 : Inport
  Action Port : ActionPort  ActionPortLabel=if(u1 < 0.5)
  Out1 : Outport
  wires:
  In1/1 -> Out1/1

== system Final_project/Delay .5s/If Action Subsystem4 ==
  In1 : Inport
  Action Port : ActionPort  ActionPortLabel=else
  Out1 : Outport
  wires:
  In1/1 -> Out1/1

== system Final_project/ATTITUDE DETERMINATION/Magnetic Sensor/NORMALIZER ==
  In1 : Inport
  Divide : Product  Inputs=*/
  Dot Product : DotProduct  InputSameDT=on  OutDataTypeStr=Inherit: Inherit via internal rule
  Sqrt : Sqrt  SaturateOnIntegerOverflow=on
  Out1 : Outport
  wires:
  Sqrt/1 -> Divide/2
  In1/1 -> Dot Product/1, Dot Product/2, Divide/1
  Dot Product/1 -> Sqrt/1
  Divide/1 -> Out1/1

== system Final_project/ATTITUDE DETERMINATION/Subsystem/Subsystem2 ==
  r_n vector : Inport
  Dot Product1 : DotProduct  InputSameDT=on  OutDataTypeStr=Inherit: Inherit via internal rule
  Sqrt1 : Sqrt  SaturateOnIntegerOverflow=on
  magnitude : Outport
  wires:
  Sqrt1/1 -> magnitude/1  "magnitude"
  Dot Product1/1 -> Sqrt1/1
  r_n vector/1 -> Dot Product1/1, Dot Product1/2

== matlab function Final_project/Approximate orbit model/MATLAB Function1 ==
  data: vector input; versor output
function versor = nromalize(vector)

versor = vector./norm(vector);

== matlab function Final_project/Approximate orbit model/MATLAB Function2 ==
  data: vector input; versor output
function versor = nromalize(vector)

versor = vector./norm(vector);

== matlab function Final_project/omega_B\L ==
  data: omegab input; omegae output; Abn input; Aln input; omegad input
function omegae = ang_vel_error(omegab,Abn,Aln,omegad)

omegae = omegab - Abn*(Aln')*omegad;

== matlab function Final_project/Magnetic torque 13th order/ECI to GEO Coord ==
  data: r_n input; lat output; t input; omega_e input; alfa_GW0 input; lon output; r output; alfa output
function [lat, lon, r, alfa] = fcn(r_n,t,omega_e,alfa_GW0)
%% Function that converts from ECEI position vector to lon, lat, radius
% INPUT:
%   r_n - position vector 
%   t - time
%   omega_e - rotational speed of earth
%   alfa_GW0 - right ascension of GW at initial time
%   alfa - LST
% OUTPUT:
%   lon - longitude from 0 to 2pi measured from the Greenwhich meridian
%   lat - latitude from -pi/2 to pi/2 measured from the equator
%   r - radius from center of earth

d = [r_n(1) r_n(2) 0];      % Projection of the position of the S/C on the 
                            % XY plane of the ECEI frame of reference
                            
alfa = acos(dot(d,[1 0 0])/norm(d));     % right ascension of the
                                         % position vector

if(d(2) < 0)
    alfa = 2*pi - alfa;

end

alfa_GW = alfa_GW0 + omega_e*t;     % RA of GW meridian at every timestep

lon = alfa - alfa_GW;               % longitude of Spacecraft
lon = mod(lon,2*pi); % wrap longitude to [0 2pi]

r = norm(r_n);

lat = asin(r_n(3)/r);   % latitude of Spacecraft

== matlab function Final_project/Magnetic torque 13th order/MATLAB Function ==
  data: X output; Y output; Z output; theta input; phi input; r input; gn input; gm input; gvali input; hn input; hm input; hvali input
function [X,Y,Z] = magnet(theta,phi,r,gn, gm, gvali,hn, hm, hvali)
% Inputs
% r     Geocentric radius
% theta Latitude measured in radians positive from equator
% phi   Longitude measured in radians positive east from Greenwich
% alfa  Right ascension
%
% Outputs - magnetic field strength in NED coordinates
% Z  B in radial direction (POSITIVE DOWN)
% X  B in NORTH direction
% Y  B in EAST direction
%
% VALIDATED ON THE BRITISH GEOLOGICAL SURVEY WEBSITE
% http://geomag.bgs.ac.uk/data_service/models_compass/igrf_calc.html


% Checks to see if located at either pole to avoid singularities
if (theta>-0.000001 && theta<0.000001)
    theta=0.000001;
elseif(theta< pi+0.000001 && theta> pi-0.000001)
    theta=pi-0.000001;
end

% Calculate the colatitude
colat = pi/2 - theta;

a=6371.2;           % Reference radius used in IGRF

N=max(gn);
g=zeros(N,N+1);
h=zeros(N,N+1);
for x=1:length(gn)
    g(gn(x),gm(x)+1) = gvali(x);
    h(hn(x),hm(x)+1) = hvali(x);
end

% Initialize each of the variables
% Br B in the radial driection
% Bt B in the colat direction
% Bp B in the phi direction


% P The associated Legendre polynomial evaluated at cos(theta)
%The nomenclature for the recursive values generally follows
% the form P10 = P(n-1,m-0)
% dP The partial derivative of P with respect to theta

Br=0;
Bt=0;
Bp=0;
P11=1;
P10=P11;
dP11=0;
dP10=dP11;
P20=0;
dP20=0;
for m=0:N
    for n=1:N
        if m<=n
            
            % Calculate Legendre polynomials and derivatives recursively
            
            if n==m
                P2 = sin(colat)*P11;
                dP2 = sin(colat)*dP11 + cos(colat)*P11;
                P11=P2;
                P10=P11;
                P20=0;
                dP11=dP2; dP10=dP11; dP20=0;
            elseif n==1
                P2 = cos(colat)*P10;
                dP2 = cos(colat)*dP10 - sin(colat)*P10;
                P20=P10;
                P10=P2;
                dP20=dP10; dP10=dP2;
            else
                K = ((n-1)^2-m^2)/((2*n-1)*(2*n-3));
                P2 = cos(colat)*P10 - K*P20;
                dP2 = cos(colat)*dP10 - sin(colat)*P10 - K*dP20;
                P20=P10;
                P10=P2;
                dP20=dP10; dP10=dP2;
            end
            % Calculate Br, Bt, and Bp
            Br = Br + (a/r)^(n+2)*(n+1)*...
                ((g(n,m+1)*cos(m*phi) + h(n,m+1)*sin(m*phi))*P2);
            Bt = Bt + (a/r)^(n+2)*...
                ((g(n,m+1)*cos(m*phi) + h(n,m+1)*sin(m*phi))*dP2);
            Bp = Bp + (a/r)^(n+2)*...
                (m*(-g(n,m+1)*sin(m*phi) + h(n,m+1)*cos(m*phi))* P2);
        end
    end
end

Z = - Br * 10^-9;
X = Bt * 10^-9;
Y = - Bp/sin(colat) *10^-9;

== matlab function Final_project/Magnetic torque 13th order/MATLAB Function2 ==
  data: a input; a output
% Link to the webpage from which the function was taken:
% http://www.leilaniphoto.com/tyson/code/wrap.m

function a = wrap(a)
% function a = wrap(a,a_center)
%
% Wraps angles to a range of 2*pi.
% Inverse of Matlab's "unwrap", and better than wrapToPi ( which has
% redundant [-pi,pi])
% Optional input "a_center" defines the center angle.  Default is 0, giving
% angles from (-pi,pi], chosen to match angle(complex(-1,0)).  Maximum
% possible value is pi.


a_center = pi;
% new way
a = mod(a,2*pi); % [0 2pi)

% shift
j = a > pi - a_center;
a(j) = a(j) - 2*pi;
j = a < a_center - pi;
a(j) = a(j) + 2*pi;

== matlab function Final_project/AERODYNAMIC DRAG TORQUE/MATLAB Function6 ==
  data: v_rel_b input; M_AERO output; rho input
function M_AERO = AERO_TORQUE(v_rel_b,rho)

%% Geometry Definition - 3U cubesat
a = 0.34;    % [m]
b = 0.1;    % [m]
c = 0.1;    % [m]

L = 0.035;      % [m] distance between center of pressure of Solar Panels and
%     centroid of the cubesat
A_SP = 0.102;   % [m^2] area of the solar panels

A = [a*b; c*b; a*c; a*b; c*b; a*c; A_SP; A_SP; A_SP; A_SP]; 

%% Physical properties definition

% Main body & solar panels
cd = 1.28;          % Drag coefficient of a flat plate


%% Main Body

% Radius of the Center of Mass wrt the centroid of the cubesat
r_CM = 0.018*[1 0 0];

% Normals to the body surfaces
n1 = [1 0 0]; n4 = -n1;
n2 = [0 1 0]; n5 = -n2;
n3 = [0 0 1]; n6 = -n3;

% radiuses wrt to the Center of mass
% ri = ri_centroid - r_CM
r1 = c/2 * n1 - r_CM; r4 = -r1;
r2 = a/2 * n2 - r_CM; r5 = -r2;
r3 = b/2 * n3 - r_CM; r6 = -r3;

%% Solar Panels
n7 = [1 0 0]; n8 = -n7;
n9 = [1 0 0]; n10 = -n9;

% radiuses wrt to the Center of mass
% ri = ri_centroid - r_CM
rSP1 = L * n2;
rSP2 = - rSP1;

%% Vector of normals
N_b = [n1; n2; n3; n4; n5; n6; n7; n8; n9; n10];

%% Vector of radiuses
R_b = [r1; r2; r3; r4; r5; r6; rSP1; rSP1; rSP2; rSP2;];

M_AERO = [0 0 0];

% Multiply by 1000 to convert from [km/s] to [m/s]
v_rel_b = v_rel_b*10^3;

for i=1:length(N_b)
    
    % Calculate the inclination to the relative velocity
    cos_i = dot(N_b(i,:),v_rel_b)/norm(v_rel_b);
    
    % Calculate the aerodinamic force on the element
    Fi = -0.5*rho*cd*norm(v_rel_b)*v_rel_b*A(i)*max(cos_i,0);
    
    % Compute the torque due to the force
    M_AERO = M_AERO + cross(R_b(i,:),Fi);
    
end

== matlab function Final_project/Approximate orbit model/orbit model - S//C orbit wrt Earth/MATLAB Function ==
  data: a input; r_vec output; e input; i input; RAAN input; omega input; f input; mu input; v_vec output
function [r_vec,v_vec] = kep2car(a,e,i,RAAN,omega,f,mu)

% Solution to: [a,e,f,RAAN,omega,i,mu]~~>[r,v]
%
% ATTENTION: 
% 1)   CHECK if it works with parabolic and hyperbolic orbits;
% PROTOTYPE:
%    [r_vec,v_vec] = kep2car(a, e, i, RAAN, omega, f, mu) 
%   
% INPUT:
%   a[1]        semi-major axis     [ km ]
%   e[1]        eccentricity        [ - ]
%   i[1]        inclination         [ rad ]
%   RAAN[1]     right ascension of the ascending node [ rad ]
%   omega[1]    argument of perigee [ rad ]
%   f[1]        true anomaly        [ rad ]
%   mu[1]      gravitational paramer [ km^3/s^2 ]
%
% OUTPUT:
%   r_vec[3]   position vector     [ km ]
%   v_vec[3]   velocity vector     [ km/s ]
%   
% CONTRIBUTORS:
%   Davide Demartini
%   Davide Iafrate
%
% VERSIONS
%   2020-10-12: First version
%   2020-11-24: Bug fixing, code cleanup
%

% Rotation Matrixes

% rotation around K of an angle RAAN

R_RAAN=[cos(RAAN)   sin(RAAN) 0
        -sin(RAAN)  cos(RAAN) 0
         0          0         1];

% rotation around the line of nodes of an angle i
R_i=[1 0 0;
    0 cos(i) sin(i)
    0 -sin(i) cos(i)]; 

% rotation around h of amount of an angle omega
R_omega=[cos(omega) sin(omega) 0
    -sin(omega) cos(omega) 0
    0 0 1]; % Perigee anomaly

% Trasformation matrix RF Perifocal ~~> Geocentric
% R = R_omega*R_i*R_RAAN  GE~~>PF
% T = R'                  PF~~>GE
T = (R_omega*R_i*R_RAAN)';

% Parameter p
p=a*(1-e^2);

% Compute position components in PF RF
r_pf = p/(1+e*cos(f));

r_pf_vect= r_pf.*[cos(f); sin(f); 0];

% Compute velocity components in PF RF

v_pf_vect= sqrt(mu/p) .* [-sin(f); (e+cos(f)); 0];

% Compute position and velocity components in Geocentric RF
% to convert vectors from the PF ref frame to the geocentric one
% we multiply the vectors in the PF frame by the matrix T
r_vec = T*r_pf_vect;
v_vec = T*v_pf_vect;

end

== matlab function Final_project/MATLAB Function4 ==
  data: S_b input; T_SRP output; F_e input; S_n input; r_n input; R_e input
function T_SRP = SRP_torque(S_b,F_e,S_n,r_n,R_e)

%% Geometry Definition - 3U cubesat
a = 0.34;    % [m]
b = 0.1;    % [m]
c = 0.1;    % [m]

L = 0.035;      % [m] distance between center of pressure of Solar Panels and
%     centroid of the cubesat
A_SP = 0.102;   % [m^2] area of the solar panels

A = [a*b; c*b; a*c; a*b; c*b; a*c; A_SP; A_SP; A_SP; A_SP]; 

%% Physical properties definition

% Main body
rho_s_MB = 0.5; rho_d_MB = 0.1;

% Solar panels
rho_s_SP = 0.8; rho_d_SP = 0.1;

%% Main Body

% Radius of the Center of Mass wrt the centroid of the cubesat
r_CM = 0.018*[1 0 0];

% Normals to the body surfaces
n1 = [1 0 0]; n4 = -n1;
n2 = [0 1 0]; n5 = -n2;
n3 = [0 0 1]; n6 = -n3;

% radiuses wrt to the Center of mass
% ri = ri_centroid - r_CM
r1 = c/2 * n1 - r_CM; r4 = -r1;
r2 = a/2 * n2 - r_CM; r5 = -r2;
r3 = b/2 * n3 - r_CM; r6 = -r3;


%% Solar Panels
n7 = [1 0 0]; n8 = -n7;
n9 = [1 0 0]; n10 = -n9;

% radiuses wrt to the Center of mass
% ri = ri_centroid - r_CM
rSP1 = L * n2;
rSP2 = - rSP1;

%% Vector of normals
N_b = [n1; n2; n3; n4; n5; n6; n7; n8; n9; n10];
%% Vector of radiuses
R_b = [r1; r2; r3; r4; r5; r6; rSP1; rSP1; rSP2; rSP2;];

%% Calculation of SRP intensity
v_c = 299792458;  % [m/s]
P = F_e / v_c;      % [N/m^2]

%% Implemented eclipse condition as shwon in Markley - Cassidis
T_SRP = [0 0 0];

S_b = S_b';

e_ES = S_n ./ norm(S_n);
if dot(r_n,e_ES) < - sqrt(norm(r_n)^2 - R_e^2)         % Sun is eclipsed by the Earth as seen by the SC
    
    T_SRP = [0 0 0];
    
else
    for i = 1:length(N_b)
        if i<= 6
            rho_s = rho_s_MB;
            rho_d = rho_d_MB;
            
        else
            rho_s = rho_s_SP;
            rho_d = rho_d_SP;
            
        end
        
        if dot(S_b,N_b(i,:))>=0
            
            F = -P*A(i)*dot(S_b,N_b(i,:))*( (1 - rho_s)*S_b + (2*rho_s*dot(S_b,N_b(i,:)) + (2/3) * rho_d).*N_b(i,:));
            T_SRP = T_SRP + cross(R_b(i,:),F);
            
        else
            T_SRP = T_SRP + [0 0 0];
        end
    end
    
    
end

== matlab function Final_project/MATLAB Function5 ==
  data: q input; q_norm output
function q_norm = normalize(q)

q_norm = q./norm(q);

== matlab function Final_project/Magnetic torque 13th order/CHECK IF IT IS CORRECT ==
  data: X input; Y input; Z input; B_ECI output; lat input; alfa input
function B_ECI = NED2ECI(X,Y,Z,lat,alfa)

% X  B in NORTH direction
% Z  B in radial direction (POSITIVE DOWN)
% Y  B in EAST direction

Bx = -(Z*cos(lat) + X*sin(lat))*cos(alfa) - Y*sin(alfa);
By = -(Z*cos(lat) + X*sin(lat))*sin(alfa) + Y*cos(alfa);
Bz = X*cos(lat) - Z*sin(lat);

B_ECI = [Bx By Bz]';

%  VALIDATED

== matlab function Final_project/ATTITUDE DETERMINATION/Magnetic Sensor/MATLAB Function ==
  data: theta input; A_epsilon output; psi input; phi input
function A_epsilon = error_matrix(theta, psi, phi)

%% Generate a random error matrix for the Sun Sensor (Lab 7)

A_epsilon = [ cos(psi)*cos(theta) cos(psi)*sin(theta)*sin(phi)+sin(psi)*cos(phi) -cos(psi)*sin(theta)*cos(phi)+sin(psi)*sin(phi)
            -sin(psi)*cos(theta)  -sin(psi)*sin(theta)*sin(phi) + cos(psi)*cos(phi) sin(psi)*sin(theta)*cos(phi) + cos(psi)*sin(phi)
            sin(theta)            -cos(theta)*sin(phi)          cos(theta)*cos(phi)];

== matlab function Final_project/ATTITUDE DETERMINATION/QUEST Attitude Determination/MATLAB Function ==
  data: B input size=[3 3]; q output size=4
function q= QUEST(B)


S = B + B';
Z = [B(2,3)-B(3,2), B(3,1)-B(1,3), B(1,2)-B(2,1)]';
sigma = trace(B);

K = [S-sigma*eye(size(S))   Z;
    Z'                      sigma;];
[V,lambda] = eig(K);
[lambda_max, i_max] = max(eig(K));
q = real(V(:,i_max));

== matlab function Final_project/CMG actuator/MATLAB Function1 ==
  data: B input; Bstar output
function Bstar = pseudoinverse(B)

Bstar = pinv(B);
